simulink model "dt_toy_model_simulation"  (R2024a)
settings: Solver=FixedStepAuto  StartTime=0.0  StopTime=Tsim  FixedStep=dT  RelTol=1e-3
values from neighbouring files (symbols this model uses):
  Ac = full(sysA)    [CT_and_DT_Controller.m]
  Ad = dt_ol_sys.A    [CT_and_DT_Controller.m]
  Bc = full(sysB)    [CT_and_DT_Controller.m]
  Bd = dt_ol_sys.B    [CT_and_DT_Controller.m]
  dt_Phiu1 = full(dt_Phiu{1})    [CT_and_DT_Controller.m]
  dt_Phiu2 = full(dt_Phiu{2})    [CT_and_DT_Controller.m]
  dt_Phiu3 = full(dt_Phiu{3})    [CT_and_DT_Controller.m]
  dt_Phiu4 = full(dt_Phiu{4})    [CT_and_DT_Controller.m]
  dt_Phiu5 = full(dt_Phiu{5})    [CT_and_DT_Controller.m]
  dt_Phiu6 = full(dt_Phiu{6})    [CT_and_DT_Controller.m]
  dt_Phiu7 = full(dt_Phiu{7})    [CT_and_DT_Controller.m]
  dt_Phix2 = full(dt_Phix{2})    [CT_and_DT_Controller.m]
  dt_Phix3 = full(dt_Phix{3})    [CT_and_DT_Controller.m]
  dt_Phix4 = full(dt_Phix{4})    [CT_and_DT_Controller.m]
  dt_Phix5 = full(dt_Phix{5})    [CT_and_DT_Controller.m]
  dt_Phix6 = full(dt_Phix{6})    [CT_and_DT_Controller.m]
  dt_Phix7 = full(dt_Phix{7})    [CT_and_DT_Controller.m]
  Ts = 0.2    [CT_and_DT_Controller.m]
  x0 = zeros(n,1)    [CT_and_DT_Controller.m]
(part 2 of 2)

== matlab function dt_toy_model_simulation/dt_SLS_gain2/z*Phi_x(z)-I/MATLAB Function3 ==
  data: u input; Mat input; y output
function y = leftMult(u,Mat)

y = Mat*u;

== matlab function dt_toy_model_simulation/OpenLoopModel1 ==
  data: Ad input; Bd input; x input; u input; delta_x output
function delta_x = dt_ss_model(Ad,Bd,x,u)
% Ad = [1.0835    0.0215    0.0002
%     0.0215    1.0623    0.0215
%     0.0002    0.0215    1.0835];
% Bd = [0.1041    0.0010    0.0000
%     0.0010    0.1031    0.0010
%     0.0000    0.0010    0.1041];

delta_x = Ad*x+Bd*u;
